simulink library "SimplusGT_2015a"  (R2015a)
settings: Solver=ode45  SolverMode=SingleTasking  StartTime=0.0  StopTime=10.0  RelTol=1e-3
undefined symbols (not defined in the file): ang_r, Cf, DiscIntNeverNeededParam, initial, Lc, Lf, m, OtherInputs, P_dc, Sbase, t0, Tm_pu, Ts, V, Vbase, w_droop, w_i, w_pll, w_tau, w_v, Wbase, wc, wfil, x0, Ybase, Zbase
libraries: powerlib x224, SimplexPS_2015a x6, SimplusGT_2015a x1
(part 4 of 5)

== system SimplusGT_2015a/Voltage Disturbance ==
  note: Model for a voltage disturbance.
      |
      | Author(s): Yitong Li
  vabc : Inport
  Controlled Voltage Source : powerlib/Electrical Sources/Controlled Voltage Source  Initialize=on  Source_Type=AC  Amplitude=0  Phase=0  Frequency=0  Measurements=None
  Controlled Voltage Source1 : powerlib/Electrical Sources/Controlled Voltage Source  Initialize=on  Source_Type=AC  Amplitude=0  Phase=0  Frequency=0  Measurements=None
  Controlled Voltage Source2 : powerlib/Electrical Sources/Controlled Voltage Source  Initialize=on  Source_Type=AC  Amplitude=0  Phase=0  Frequency=0  Measurements=None
  Demux : Demux  Outputs=3
  Gain : Gain  Gain=Vbase
  a+ : PMIOPort  Side=Right
  a- : PMIOPort  Port=2  Side=Left
  b+ : PMIOPort  Port=3  Side=Right
  b- : PMIOPort  Port=4  Side=Left
  c+ : PMIOPort  Port=5  Side=Right
  c- : PMIOPort  Port=6  Side=Left
  wires:
  vabc/1 -> Gain/1
  Demux/1 -> Controlled Voltage Source/1
  Demux/2 -> Controlled Voltage Source1/1
  Demux/3 -> Controlled Voltage Source2/1
  Gain/1 -> Demux/1
  connections:
  Controlled Voltage Source2/LConn1 -- c-/RConn1
  Controlled Voltage Source1/RConn1 -- b+/RConn1
  Controlled Voltage Source2/RConn1 -- c+/RConn1
  Controlled Voltage Source/RConn1 -- a+/RConn1
  Controlled Voltage Source/LConn1 -- a-/RConn1
  Controlled Voltage Source1/LConn1 -- b-/RConn1

== system SimplusGT_2015a/abc -> alpha//beta (Power-Invariant) ==
  note: Frame transformation from abc to alpha/beta.
      |
      | Author(s): Yitong Li
      |
      | Notes:
      |
      | The transformation is power-invariant.
  abc : Inport
  ->alpha : Fcn  Expr=u(1) - 1/2*u(2) - 1/2*u(3)
  ->beta : Fcn  Expr=0 + sqrt(3)/2*u(2) - sqrt(3)/2*u(3)
  Gain : Gain  Gain=sqrt(2/3)
  Mux2 : Mux  Inputs=2
  albe : Outport
  wires:
  abc/1 -> Gain/1
  Mux2/1 -> albe/1
  Gain/1 -> ->alpha/1, ->beta/1
  ->alpha/1 -> Mux2/1
  ->beta/1 -> Mux2/2

== system SimplusGT_2015a/abc -> alpha//beta//0 (Power-Invariant) ==
  note: Frame transformation from abc to alpha/beta/0.
      |
      | Author(s): Yitong Li
      |
      | Notes:
      |
      | The transformation is power-invariant.
  abc : Inport
  ->0 : Fcn  Expr=1/sqrt(2)*u(1) + 1/sqrt(2)*u(2) + 1/sqrt(2)*u(3)
  ->alpha : Fcn  Expr=u(1) - 1/2*u(2) - 1/2*u(3)
  ->beta : Fcn  Expr=0 + sqrt(3)/2*u(2) - sqrt(3)/2*u(3)
  Gain : Gain  Gain=sqrt(2/3)
  Mux2 : Mux  Inputs=3
  albe0 : Outport
  wires:
  ->beta/1 -> Mux2/2
  ->alpha/1 -> Mux2/1
  Gain/1 -> ->alpha/1, ->0/1, ->beta/1
  Mux2/1 -> albe0/1
  abc/1 -> Gain/1
  ->0/1 -> Mux2/3

== system SimplusGT_2015a/abc -> dq (Power-Invariant) ==
  note: Frame transformation from abc to dq.
      |
      | Author(s): Yitong Li
      |
      | Notes:
      |
      | The transformation is power-invariant.
      |
      | theta is the angle that d axis leads a axis.
      |
      | q axis leads d axis by 90 degrees.
  abc : Inport
  theta : Inport  Port=2
  ->d : Fcn  Expr=cos(u(4))*u(1) + cos(u(4)-2/3*pi)*u(2) + cos(u(4)-4/3*pi)*u(3)
  ->q : Fcn  Expr=-sin(u(4))*u(1) - sin(u(4)-2/3*pi)*u(2) - sin(u(4)-4/3*pi)*u(3)
  Gain : Gain  Gain=sqrt(2/3)
  Mux5 : Mux  Inputs=2
  Mux6 : Mux  Inputs=2
  dq : Outport
  wires:
  Mux5/1 -> ->q/1, ->d/1
  Mux6/1 -> dq/1
  ->q/1 -> Mux6/2
  theta/1 -> Mux5/2
  Gain/1 -> Mux5/1
  ->d/1 -> Mux6/1
  abc/1 -> Gain/1

== system SimplusGT_2015a/abc -> dq (Power-Invariant) (Complex Theta) ==
  abc : Inport
  theta+ : Inport  Port=2
  ->d : Fcn  Expr=cos(u(4))*u(1) + cos(u(4)-2/3*pi)*u(2) + cos(u(4)-4/3*pi)*u(3)
  ->q : Fcn  Expr=-sin(u(4))*u(1) - sin(u(4)-2/3*pi)*u(2) - sin(u(4)-4/3*pi)*u(3)
  Complex to Real-Imag : ComplexToRealImag
  Gain : Gain  Gain=sqrt(2/3)
  Math Function : Math  SaturateOnIntegerOverflow=on
  Mux5 : Mux  Inputs=2
  Mux6 : Mux  Inputs=2
  Product : Product
  dq : Outport
  wires:
  ->q/1 -> Mux6/2
  abc/1 -> Gain/1
  Mux5/1 -> ->q/1, ->d/1
  Mux6/1 -> dq/1
  ->d/1 -> Mux6/1
  theta+/1 -> Complex to Real-Imag/1
  Complex to Real-Imag/1 -> Mux5/2
  Complex to Real-Imag/2 -> Math Function/1
  Gain/1 -> Product/1
  Product/1 -> Mux5/1
  Math Function/1 -> Product/2

== system SimplusGT_2015a/abc -> dq0 (Power-Invariant) ==
  note: Frame transformation from abc to dq0.
      |
      | Author(s): Yitong Li
      |
      | Notes:
      |
      | The transformation is power-invariant.
      |
      | theta is the angle that dq axis leads abc axis, specifically, d axis leads a axis.
      |
      | q axis leads d axis by 90 degrees. b leads a axis 90 degrees. c leads b 90 degrees.
  abc : Inport
  theta : Inport  Port=2
  ->0 : Fcn  Expr=sqrt(2)/2*u(1) + sqrt(2)/2*u(2) + sqrt(2)/2*u(3)
  ->d : Fcn  Expr=cos(u(4))*u(1) + cos(u(4)-2/3*pi)*u(2) + cos(u(4)-4/3*pi)*u(3)
  ->q : Fcn  Expr=-sin(u(4))*u(1) - sin(u(4)-2/3*pi)*u(2) - sin(u(4)-4/3*pi)*u(3)
  Gain : Gain  Gain=sqrt(2/3)
  Mux1 : Mux  Inputs=2
  Mux2 : Mux  Inputs=3
  dq0 : Outport
  wires:
  ->d/1 -> Mux2/1
  ->q/1 -> Mux2/2
  Gain/1 -> Mux1/1
  abc/1 -> Gain/1
  theta/1 -> Mux1/2
  Mux1/1 -> ->0/1, ->d/1, ->q/1
  Mux2/1 -> dq0/1
  ->0/1 -> Mux2/3

== system SimplusGT_2015a/abc->dq (Power-Invariant) (theta_dq) ==
  abc : Inport
  theta_dq : Inport  Port=2
  ->d : Fcn  Expr=cos(u(4))*u(1) + cos(u(4)-2/3*pi)*u(2) + cos(u(4)-4/3*pi)*u(3)
  ->q : Fcn  Expr=-sin(u(4))*u(1) - sin(u(4)-2/3*pi)*u(2) - sin(u(4)-4/3*pi)*u(3)
  Demux : Demux  Outputs=2
  Gain : Gain  Gain=sqrt(2/3)
  Math Function : Math  SaturateOnIntegerOverflow=on
  Mux5 : Mux  Inputs=2
  Mux6 : Mux  Inputs=2
  Product : Product
  dq : Outport
  wires:
  Gain/1 -> Product/1
  Math Function/1 -> Product/2
  Mux6/1 -> dq/1
  Mux5/1 -> ->q/1, ->d/1
  ->d/1 -> Mux6/1
  Product/1 -> Mux5/1
  abc/1 -> Gain/1
  ->q/1 -> Mux6/2
  theta_dq/1 -> Demux/1
  Demux/1 -> Mux5/2
  Demux/2 -> Math Function/1

== system SimplusGT_2015a/alpha//beta -> abc (Power-Invariant) ==
  note: Frame transformation from alpha/beta to abc.
      |
      | Author(s): Yitong Li
      |
      | Notes:
      |
      | The transformation is power-invariant.
  albe : Inport
  ->a : Fcn  Expr=u(1) + 0
  ->b : Fcn  Expr=-1/2*u(1) + sqrt(3)/2*u(2)
  ->c : Fcn  Expr=-1/2*u(1) - sqrt(3)/2*u(2)
  Gain : Gain  Gain=sqrt(2/3)
  Mux2 : Mux  Inputs=3
  abc : Outport
  wires:
  Gain/1 -> ->a/1, ->c/1, ->b/1
  Mux2/1 -> abc/1
  ->c/1 -> Mux2/3
  ->b/1 -> Mux2/2
  ->a/1 -> Mux2/1
  albe/1 -> Gain/1

== system SimplusGT_2015a/alpha//beta -> dq ==
  note: Frame transformation from alpha/beta to dq.
      |
      | Author(s): Yitong Li
      |
      | Notes:
      |
      | theta is the angle that dq axis leads alpha/beta axis, specifically, d axis leads alpha axis.
  albe : Inport
  theta : Inport  Port=2
  ->d : Fcn  Expr=cos(u(3))*u(1) + sin(u(3))*u(2)
  ->q : Fcn  Expr=-sin(u(3))*u(1) + cos(u(3))*u(2)
  Mux5 : Mux  Inputs=2
  Mux6 : Mux  Inputs=2
  dq : Outport
  wires:
  Mux5/1 -> ->q/1, ->d/1
  albe/1 -> Mux5/1
  theta/1 -> Mux5/2
  Mux6/1 -> dq/1
  ->q/1 -> Mux6/2
  ->d/1 -> Mux6/1

== system SimplusGT_2015a/alpha//beta//0 -> abc (Power-Invariant) ==
  note: Frame transformation from alpha/beta0 to abc.
      |
      | Author(s): Yitong Li
      |
      | Notes:
      |
      | The transformation is power-invariant.
  albe0 : Inport
  ->a : Fcn  Expr=u(1) + 0 + 1/sqrt(2)*u(3)
  ->b : Fcn  Expr=-1/2*u(1) + sqrt(3)/2*u(2) + 1/sqrt(2)*u(3)
  ->c : Fcn  Expr=-1/2*u(1) - sqrt(3)/2*u(2) + 1/sqrt(2)*u(3)
  Gain : Gain  Gain=sqrt(2/3)
  Mux2 : Mux  Inputs=3
  abc : Outport
  wires:
  Gain/1 -> ->a/1, ->c/1, ->b/1
  ->c/1 -> Mux2/3
  albe0/1 -> Gain/1
  ->a/1 -> Mux2/1
  ->b/1 -> Mux2/2
  Mux2/1 -> abc/1

== system SimplusGT_2015a/dq -> abc (Power-Invariant) ==
  note: Frame transformation from dq to abc.
      |
      | Author(s): Yitong Li
      |
      | Notes:
      |
      | The transformation is power-invariant.
      |
      | theta is the angle that dq axis leads alpha/beta axis, specifically, d axis leads alpha axis.
  dq : Inport
  theta : Inport  Port=2
  ->a : Fcn  Expr=cos(u(3))*u(1) - sin(u(3))*u(2)
  ->b : Fcn  Expr=cos(u(3)-2/3*pi)*u(1) - sin(u(3)-2/3*pi)*u(2)
  ->c : Fcn  Expr=cos(u(3)-4/3*pi)*u(1) - sin(u(3)-4/3*pi)*u(2)
  Gain : Gain  Gain=sqrt(2/3)
  Mux5 : Mux  Inputs=2
  Mux6 : Mux  Inputs=3
  abc : Outport
  wires:
  theta/1 -> Mux5/2
  Mux5/1 -> ->c/1, ->a/1, ->b/1
  Mux6/1 -> abc/1
  ->c/1 -> Mux6/3
  dq/1 -> Gain/1
  Gain/1 -> Mux5/1
  ->a/1 -> Mux6/1
  ->b/1 -> Mux6/2

== system SimplusGT_2015a/dq -> abc (Power-Invariant) (Complex Theta) ==
  dq : Inport
  theta+ : Inport  Port=2
  ->a : Fcn  Expr=cos(u(3))*u(1) - sin(u(3))*u(2)
  ->b : Fcn  Expr=cos(u(3)-2/3*pi)*u(1) - sin(u(3)-2/3*pi)*u(2)
  ->c : Fcn  Expr=cos(u(3)-4/3*pi)*u(1) - sin(u(3)-4/3*pi)*u(2)
  Complex to Real-Imag : ComplexToRealImag
  Gain : Gain  Gain=sqrt(2/3)
  Gain1 : Gain  Gain=-1
  Math Function : Math  SaturateOnIntegerOverflow=on
  Mux5 : Mux  Inputs=2
  Mux6 : Mux  Inputs=3
  Product : Product
  abc : Outport
  wires:
  ->b/1 -> Mux6/2
  ->a/1 -> Mux6/1
  dq/1 -> Gain/1
  ->c/1 -> Mux6/3
  Mux6/1 -> abc/1
  Mux5/1 -> ->c/1, ->a/1, ->b/1
  theta+/1 -> Complex to Real-Imag/1
  Math Function/1 -> Product/2
  Complex to Real-Imag/1 -> Mux5/2
  Product/1 -> Mux5/1
  Gain/1 -> Product/1
  Complex to Real-Imag/2 -> Gain1/1
  Gain1/1 -> Math Function/1

== system SimplusGT_2015a/dq->abc (Power-Invariant) (theta_dq) ==
  dq : Inport
  theta_dq : Inport  Port=2
  ->a : Fcn  Expr=cos(u(3))*u(1) - sin(u(3))*u(2)
  ->b : Fcn  Expr=cos(u(3)-2/3*pi)*u(1) - sin(u(3)-2/3*pi)*u(2)
  ->c : Fcn  Expr=cos(u(3)-4/3*pi)*u(1) - sin(u(3)-4/3*pi)*u(2)
  Demux : Demux  Outputs=2
  Gain : Gain  Gain=sqrt(2/3)
  Gain1 : Gain  Gain=-1
  Math Function : Math  SaturateOnIntegerOverflow=on
  Mux5 : Mux  Inputs=2
  Mux6 : Mux  Inputs=3
  Product : Product
  abc : Outport
  wires:
  Mux6/1 -> abc/1
  Demux/1 -> Mux5/2
  Product/1 -> Mux5/1
  ->a/1 -> Mux6/1
  Gain1/1 -> Math Function/1
  Math Function/1 -> Product/2
  ->c/1 -> Mux6/3
  Mux5/1 -> ->c/1, ->a/1, ->b/1
  ->b/1 -> Mux6/2
  theta_dq/1 -> Demux/1
  Gain/1 -> Product/1
  dq/1 -> Gain/1
  Demux/2 -> Gain1/1

== system SimplusGT_2015a/dq0 -> abc (Power-Invariant) ==
  note: Frame transformation from dq0 to abc.
      |
      | Author(s): Yitong Li
      |
      | Notes:
      |
      | The transformation is power-invariant.
      |
      | theta is the angle that dq axis leads alpha/beta axis, specifically, d axis leads alpha axis.
  dq0 : Inport
  theta : Inport  Port=2
  ->a : Fcn  Expr=cos(u(4))*u(1) - sin(u(4))*u(2) + sqrt(2)/2*u(3)
  ->b : Fcn  Expr=cos(u(4)-2/3*pi)*u(1) - sin(u(4)-2/3*pi)*u(2) + sqrt(2)/2*u(3)
  ->c : Fcn  Expr=cos(u(4)-4/3*pi)*u(1) - sin(u(4)-4/3*pi)*u(2) + sqrt(2)/2*u(3)
  Gain : Gain  Gain=sqrt(2/3)
  Mux1 : Mux  Inputs=2
  Mux2 : Mux  Inputs=3
  abc : Outport
  wires:
  ->a/1 -> Mux2/1
  ->b/1 -> Mux2/2
  Gain/1 -> Mux1/1
  dq0/1 -> Gain/1
  theta/1 -> Mux1/2
  Mux1/1 -> ->c/1, ->a/1, ->b/1
  Mux2/1 -> abc/1
  ->c/1 -> Mux2/3

== system SimplusGT_2015a/x1y1 -> x2y2 ==
  note: Frame transformation from x1y1 to x2y2.
      |
      | Author(s): Yitong Li
      |
      | Notes:
      |
      | theta is the phase angle that coordinate 2 (axis) leads coordinate 1 (axis).
  x1y1 : Inport
  theta : Inport  Port=2
  ->x2 : Fcn  Expr=cos(u(3))*u(1) + sin(u(3))*u(2)
  ->y2 : Fcn  Expr=-sin(u(3))*u(1) + cos(u(3))*u(2)
  Mux5 : Mux  Inputs=2
  Mux6 : Mux  Inputs=2
  x2y2 : Outport
  wires:
  Mux6/1 -> x2y2/1
  Mux5/1 -> ->y2/1, ->x2/1
  theta/1 -> Mux5/2
  x1y1/1 -> Mux5/1
  ->y2/1 -> Mux6/2
  ->x2/1 -> Mux6/1

== system SimplusGT_2015a/x2y2 -> x1y1 ==
  note: Frame transformation from x2y2 to x1y1.
      |
      | Author(s): Yitong Li
      |
      | Notes:
      |
      | theta is the phase angle that coordinate 2 (axis) leads coordinate 1 (axis).
  x2y2 : Inport
  theta : Inport  Port=2
  ->x2 : Fcn  Expr=cos(u(3))*u(1) - sin(u(3))*u(2)
  ->y2 : Fcn  Expr=sin(u(3))*u(1) + cos(u(3))*u(2)
  Mux5 : Mux  Inputs=2
  Mux6 : Mux  Inputs=2
  x1y1 : Outport
  wires:
  theta/1 -> Mux5/2
  Mux6/1 -> x1y1/1
  Mux5/1 -> ->y2/1, ->x2/1
  x2y2/1 -> Mux5/1
  ->x2/1 -> Mux6/1
  ->y2/1 -> Mux6/2

== system SimplusGT_2015a/AC Infinite Bus (Current Type)/PQ Calculation (dq-Frame) ==
  note: Power calculation.
      |
      | Author(s): Yitong Li
      |
      | Notes:
      |
      | The calculation is done in dq frame.
  vdq : Inport
  idq : Inport  Port=2
  Mux : Mux  Inputs=2
  Mux1 : Mux  Inputs=2
  P = vd*id+vq*iq : Fcn  Expr=u[1]*u[3]+u[2]*u[4]
  Q = -vd*iq+vq*id : Fcn  Expr=-u[1]*u[4]+u[2]*u[3]
  pq : Outport
  wires:
  Q = -vd*iq+vq*id/1 -> Mux/2
  Mux1/1 -> Q = -vd*iq+vq*id/1, P = vd*id+vq*iq/1
  idq/1 -> Mux1/2
  vdq/1 -> Mux1/1
  P = vd*id+vq*iq/1 -> Mux/1
  Mux/1 -> pq/1

== system SimplusGT_2015a/AC Infinite Bus (Current Type)/abc -> dq (Power-Invariant) ==
  note: Frame transformation from abc to dq.
      |
      | Author(s): Yitong Li
      |
      | Notes:
      |
      | The transformation is power-invariant.
      |
      | theta is the angle that d axis leads a axis.
      |
      | q axis leads d axis by 90 degrees.
  abc : Inport
  theta : Inport  Port=2
  ->d : Fcn  Expr=cos(u(4))*u(1) + cos(u(4)-2/3*pi)*u(2) + cos(u(4)-4/3*pi)*u(3)
  ->q : Fcn  Expr=-sin(u(4))*u(1) - sin(u(4)-2/3*pi)*u(2) - sin(u(4)-4/3*pi)*u(3)
  Gain : Gain  Gain=sqrt(2/3)
  Mux5 : Mux  Inputs=2
  Mux6 : Mux  Inputs=2
  dq : Outport
  wires:
  Mux5/1 -> ->q/1, ->d/1
  Mux6/1 -> dq/1
  ->q/1 -> Mux6/2
  theta/1 -> Mux5/2
  Gain/1 -> Mux5/1
  ->d/1 -> Mux6/1
  abc/1 -> Gain/1

== system SimplusGT_2015a/AC Infinite Bus (Current Type)/dq -> abc (Power-Invariant) ==
  note: Frame transformation from dq to abc.
      |
      | Author(s): Yitong Li
      |
      | Notes:
      |
      | The transformation is power-invariant.
      |
      | theta is the angle that dq axis leads alpha/beta axis, specifically, d axis leads alpha axis.
  dq : Inport
  theta : Inport  Port=2
  ->a : Fcn  Expr=cos(u(3))*u(1) - sin(u(3))*u(2)
  ->b : Fcn  Expr=cos(u(3)-2/3*pi)*u(1) - sin(u(3)-2/3*pi)*u(2)
  ->c : Fcn  Expr=cos(u(3)-4/3*pi)*u(1) - sin(u(3)-4/3*pi)*u(2)
  Gain : Gain  Gain=sqrt(2/3)
  Mux5 : Mux  Inputs=2
  Mux6 : Mux  Inputs=3
  abc : Outport
  wires:
  theta/1 -> Mux5/2
  Mux5/1 -> ->c/1, ->a/1, ->b/1
  Mux6/1 -> abc/1
  ->c/1 -> Mux6/3
  dq/1 -> Gain/1
  Gain/1 -> Mux5/1
  ->a/1 -> Mux6/1
  ->b/1 -> Mux6/2

== system SimplusGT_2015a/AC Infinite Bus (Voltage Type)/PQ Calculation (dq-Frame)1 ==
  note: Power calculation.
      |
      | Author(s): Yitong Li
      |
      | Notes:
      |
      | The calculation is done in dq frame.
  vdq : Inport
  idq : Inport  Port=2
  Mux : Mux  Inputs=2
  Mux1 : Mux  Inputs=2
  P = vd*id+vq*iq : Fcn  Expr=u[1]*u[3]+u[2]*u[4]
  Q = -vd*iq+vq*id : Fcn  Expr=-u[1]*u[4]+u[2]*u[3]
  pq : Outport
  wires:
  Q = -vd*iq+vq*id/1 -> Mux/2
  Mux1/1 -> Q = -vd*iq+vq*id/1, P = vd*id+vq*iq/1
  idq/1 -> Mux1/2
  vdq/1 -> Mux1/1
  P = vd*id+vq*iq/1 -> Mux/1
  Mux/1 -> pq/1

== system SimplusGT_2015a/AC Infinite Bus (Voltage Type)/abc -> dq (Power-Invariant)1 ==
  note: Frame transformation from abc to dq.
      |
      | Author(s): Yitong Li
      |
      | Notes:
      |
      | The transformation is power-invariant.
      |
      | theta is the angle that d axis leads a axis.
      |
      | q axis leads d axis by 90 degrees.
  abc : Inport
  theta : Inport  Port=2
  ->d : Fcn  Expr=cos(u(4))*u(1) + cos(u(4)-2/3*pi)*u(2) + cos(u(4)-4/3*pi)*u(3)
  ->q : Fcn  Expr=-sin(u(4))*u(1) - sin(u(4)-2/3*pi)*u(2) - sin(u(4)-4/3*pi)*u(3)
  Gain : Gain  Gain=sqrt(2/3)
  Mux5 : Mux  Inputs=2
  Mux6 : Mux  Inputs=2
  dq : Outport
  wires:
  Mux5/1 -> ->q/1, ->d/1
  Mux6/1 -> dq/1
  ->q/1 -> Mux6/2
  theta/1 -> Mux5/2
  Gain/1 -> Mux5/1
  ->d/1 -> Mux6/1
  abc/1 -> Gain/1

== system SimplusGT_2015a/AC Infinite Bus (Voltage Type)/dq -> abc (Power-Invariant)1 ==
  note: Frame transformation from dq to abc.
      |
      | Author(s): Yitong Li
      |
      | Notes:
      |
      | The transformation is power-invariant.
      |
      | theta is the angle that dq axis leads alpha/beta axis, specifically, d axis leads alpha axis.
  dq : Inport
  theta : Inport  Port=2
  ->a : Fcn  Expr=cos(u(3))*u(1) - sin(u(3))*u(2)
  ->b : Fcn  Expr=cos(u(3)-2/3*pi)*u(1) - sin(u(3)-2/3*pi)*u(2)
  ->c : Fcn  Expr=cos(u(3)-4/3*pi)*u(1) - sin(u(3)-4/3*pi)*u(2)
  Gain : Gain  Gain=sqrt(2/3)
  Mux5 : Mux  Inputs=2
  Mux6 : Mux  Inputs=3
  abc : Outport
  wires:
  theta/1 -> Mux5/2
  Mux5/1 -> ->c/1, ->a/1, ->b/1
  Mux6/1 -> abc/1
  ->c/1 -> Mux6/3
  dq/1 -> Gain/1
  Gain/1 -> Mux5/1
  ->a/1 -> Mux6/1
  ->b/1 -> Mux6/2

== system SimplusGT_2015a/Frequency Droop (iDQ -> id)/x1y1 -> x2y2 ==
  note: Frame transformation from x1y1 to x2y2.
      |
      | Author(s): Yitong Li
      |
      | Notes:
      |
      | theta is the phase angle that coordinate 2 (axis) leads coordinate 1 (axis).
  x1y1 : Inport
  theta : Inport  Port=2
  ->x2 : Fcn  Expr=cos(u(3))*u(1) + sin(u(3))*u(2)
  ->y2 : Fcn  Expr=-sin(u(3))*u(1) + cos(u(3))*u(2)
  Mux5 : Mux  Inputs=2
  Mux6 : Mux  Inputs=2
  x2y2 : Outport
  wires:
  ->x2/1 -> Mux6/1
  ->y2/1 -> Mux6/2
  x1y1/1 -> Mux5/1
  theta/1 -> Mux5/2
  Mux5/1 -> ->x2/1, ->y2/1
  Mux6/1 -> x2y2/1

== system SimplusGT_2015a/Frequency Droop (iabc -> id)/abc -> dq (Power-Invariant) ==
  note: Frame transformation from abc to dq.
      |
      | Author(s): Yitong Li
      |
      | Notes:
      |
      | The transformation is power-invariant.
      |
      | theta is the angle that d axis leads a axis.
      |
      | q axis leads d axis by 90 degrees.
  abc : Inport
  theta : Inport  Port=2
  ->d : Fcn  Expr=cos(u(4))*u(1) + cos(u(4)-2/3*pi)*u(2) + cos(u(4)-4/3*pi)*u(3)
  ->q : Fcn  Expr=-sin(u(4))*u(1) - sin(u(4)-2/3*pi)*u(2) - sin(u(4)-4/3*pi)*u(3)
  Gain : Gain  Gain=sqrt(2/3)
  Mux5 : Mux  Inputs=2
  Mux6 : Mux  Inputs=2
  dq : Outport
  wires:
  abc/1 -> Gain/1
  ->d/1 -> Mux6/1
  Gain/1 -> Mux5/1
  theta/1 -> Mux5/2
  ->q/1 -> Mux6/2
  Mux6/1 -> dq/1
  Mux5/1 -> ->d/1, ->q/1

== system SimplusGT_2015a/Frequency Droop (iabc -> id+jiq)/abc -> dq (Power-Invariant)1 ==
  note: Frame transformation from abc to dq.
      |
      | Author(s): Yitong Li
      |
      | Notes:
      |
      | The transformation is power-invariant.
      |
      | theta is the angle that d axis leads a axis.
      |
      | q axis leads d axis by 90 degrees.
  abc : Inport
  theta : Inport  Port=2
  ->d : Fcn  Expr=cos(u(4))*u(1) + cos(u(4)-2/3*pi)*u(2) + cos(u(4)-4/3*pi)*u(3)
  ->q : Fcn  Expr=-sin(u(4))*u(1) - sin(u(4)-2/3*pi)*u(2) - sin(u(4)-4/3*pi)*u(3)
  Gain : Gain  Gain=sqrt(2/3)
  Mux5 : Mux  Inputs=2
  Mux6 : Mux  Inputs=2
  dq : Outport
  wires:
  abc/1 -> Gain/1
  ->d/1 -> Mux6/1
  Gain/1 -> Mux5/1
  theta/1 -> Mux5/2
  ->q/1 -> Mux6/2
  Mux6/1 -> dq/1
  Mux5/1 -> ->d/1, ->q/1

== system SimplusGT_2015a/Frequency Droop (iabc -> iq)/abc -> dq (Power-Invariant)1 ==
  note: Frame transformation from abc to dq.
      |
      | Author(s): Yitong Li
      |
      | Notes:
      |
      | The transformation is power-invariant.
      |
      | theta is the angle that d axis leads a axis.
      |
      | q axis leads d axis by 90 degrees.
  abc : Inport
  theta : Inport  Port=2
  ->d : Fcn  Expr=cos(u(4))*u(1) + cos(u(4)-2/3*pi)*u(2) + cos(u(4)-4/3*pi)*u(3)
  ->q : Fcn  Expr=-sin(u(4))*u(1) - sin(u(4)-2/3*pi)*u(2) - sin(u(4)-4/3*pi)*u(3)
  Gain : Gain  Gain=sqrt(2/3)
  Mux5 : Mux  Inputs=2
  Mux6 : Mux  Inputs=2
  dq : Outport
  wires:
  abc/1 -> Gain/1
  ->d/1 -> Mux6/1
  Gain/1 -> Mux5/1
  theta/1 -> Mux5/2
  ->q/1 -> Mux6/2
  Mux6/1 -> dq/1
  Mux5/1 -> ->d/1, ->q/1

== system SimplusGT_2015a/Grid-Following Voltage-Source Inverter (dq-Frame System Object)/PQ Calculation (dq-Frame)1 ==
  note: Power calculation.
      |
      | Author(s): Yitong Li
      |
      | Notes:
      |
      | The calculation is done in dq frame.
  vdq : Inport
  idq : Inport  Port=2
  Mux : Mux  Inputs=2
  Mux1 : Mux  Inputs=2
  P = vd*id+vq*iq : Fcn  Expr=u[1]*u[3]+u[2]*u[4]
  Q = -vd*iq+vq*id : Fcn  Expr=-u[1]*u[4]+u[2]*u[3]
  pq : Outport
  wires:
  Q = -vd*iq+vq*id/1 -> Mux/2
  Mux1/1 -> Q = -vd*iq+vq*id/1, P = vd*id+vq*iq/1
  idq/1 -> Mux1/2
  vdq/1 -> Mux1/1
  P = vd*id+vq*iq/1 -> Mux/1
  Mux/1 -> pq/1

== system SimplusGT_2015a/Grid-Following Voltage-Source Inverter (dq-Frame System Object)/abc -> dq (Power-Invariant)1 ==
  note: Frame transformation from abc to dq.
      |
      | Author(s): Yitong Li
      |
      | Notes:
      |
      | The transformation is power-invariant.
      |
      | theta is the angle that d axis leads a axis.
      |
      | q axis leads d axis by 90 degrees.
  abc : Inport
  theta : Inport  Port=2
  ->d : Fcn  Expr=cos(u(4))*u(1) + cos(u(4)-2/3*pi)*u(2) + cos(u(4)-4/3*pi)*u(3)
  ->q : Fcn  Expr=-sin(u(4))*u(1) - sin(u(4)-2/3*pi)*u(2) - sin(u(4)-4/3*pi)*u(3)
  Gain : Gain  Gain=sqrt(2/3)
  Mux5 : Mux  Inputs=2
  Mux6 : Mux  Inputs=2
  dq : Outport
  wires:
  Mux5/1 -> ->q/1, ->d/1
  Mux6/1 -> dq/1
  ->q/1 -> Mux6/2
  theta/1 -> Mux5/2
  Gain/1 -> Mux5/1
  ->d/1 -> Mux6/1
  abc/1 -> Gain/1

== system SimplusGT_2015a/Grid-Following Voltage-Source Inverter (dq-Frame System Object)/abc -> dq (Power-Invariant)2 ==
  note: Frame transformation from abc to dq.
      |
      | Author(s): Yitong Li
      |
      | Notes:
      |
      | The transformation is power-invariant.
      |
      | theta is the angle that d axis leads a axis.
      |
      | q axis leads d axis by 90 degrees.
  abc : Inport
  theta : Inport  Port=2
  ->d : Fcn  Expr=cos(u(4))*u(1) + cos(u(4)-2/3*pi)*u(2) + cos(u(4)-4/3*pi)*u(3)
  ->q : Fcn  Expr=-sin(u(4))*u(1) - sin(u(4)-2/3*pi)*u(2) - sin(u(4)-4/3*pi)*u(3)
  Gain : Gain  Gain=sqrt(2/3)
  Mux5 : Mux  Inputs=2
  Mux6 : Mux  Inputs=2
  dq : Outport
  wires:
  Mux5/1 -> ->q/1, ->d/1
  Mux6/1 -> dq/1
  ->q/1 -> Mux6/2
  theta/1 -> Mux5/2
  Gain/1 -> Mux5/1
  ->d/1 -> Mux6/1
  abc/1 -> Gain/1

== system SimplusGT_2015a/Grid-Following Voltage-Source Inverter (dq-Frame System Object)/dq -> abc (Power-Invariant)1 ==
  note: Frame transformation from dq to abc.
      |
      | Author(s): Yitong Li
      |
      | Notes:
      |
      | The transformation is power-invariant.
      |
      | theta is the angle that dq axis leads alpha/beta axis, specifically, d axis leads alpha axis.
  dq : Inport
  theta : Inport  Port=2
  ->a : Fcn  Expr=cos(u(3))*u(1) - sin(u(3))*u(2)
  ->b : Fcn  Expr=cos(u(3)-2/3*pi)*u(1) - sin(u(3)-2/3*pi)*u(2)
  ->c : Fcn  Expr=cos(u(3)-4/3*pi)*u(1) - sin(u(3)-4/3*pi)*u(2)
  Gain : Gain  Gain=sqrt(2/3)
  Mux5 : Mux  Inputs=2
  Mux6 : Mux  Inputs=3
  abc : Outport
  wires:
  theta/1 -> Mux5/2
  Mux5/1 -> ->c/1, ->a/1, ->b/1
  Mux6/1 -> abc/1
  ->c/1 -> Mux6/3
  dq/1 -> Gain/1
  Gain/1 -> Mux5/1
  ->a/1 -> Mux6/1
  ->b/1 -> Mux6/2

== system SimplusGT_2015a/Grid-Following Inverter (Simulink Block)/Current Controller ==
  iIdq* : Inport
  iIdq : Inport  Port=2
  vdq : Inport  Port=3
  enable : Inport  Port=4
  Constant : Constant  Value=Kcd
  Demux1 : Demux  Outputs=2
  Demux2 : Demux  Outputs=2
  Demux3 : Demux  Outputs=2
  Mux : Mux  Inputs=2
  PI-DT-Estimated d : Subsystem  mask{Lf=Lf, Kg=Kg, Kp=Kp, Ki=Ki, xmax=vdmax, xmin=-vdmax, Ts=Ts}
      mask prompts: Lf "Inductance"; Kg "Estimator Gain"; Kp "Proportional Gain"; Ki "Integral Gain"; xmax "Upper Limit"; xmin "Lower Limit"; Ts "Sampling Time"
  PI-DT-Estimated q : Subsystem  mask{Lf=Lf, Kg=Kg, Kp=Kp, Ki=Ki, xmax=vqmax, xmin=-vqmax, Ts=Ts}
      mask prompts: Lf "Inductance"; Kg "Estimator Gain"; Kp "Proportional Gain"; Ki "Integral Gain"; xmax "Upper Limit"; xmin "Lower Limit"; Ts "Sampling Time"
  Product : Product
  Product1 : Product
  sum_d : Sum  Inputs=+-
  sum_q : Sum
  wLd : Gain  Gain=Wbase*Lf
  wLq : Gain  Gain=Wbase*Lf
  vidq* : Outport
  wires:
  sum_d/1 -> Mux/1
  sum_q/1 -> Mux/2
  iIdq/1 -> Demux1/1
  Demux1/1 -> wLd/1, PI-DT-Estimated d/4(actual)
  Demux1/2 -> PI-DT-Estimated q/1(actual), wLq/1
  Mux/1 -> vidq*/1
  PI-DT-Estimated d/1(Out) -> sum_d/1
  vdq/1 -> Demux3/1
  PI-DT-Estimated q/1(Out) -> sum_q/2
  Demux3/2 -> PI-DT-Estimated q/2(initial)
  Demux3/1 -> PI-DT-Estimated d/3(initial)
  iIdq*/1 -> Demux2/1
  Demux2/1 -> PI-DT-Estimated d/2(reference)
  Demux2/2 -> PI-DT-Estimated q/3(reference)
  enable/1 -> PI-DT-Estimated q/4(enable), PI-DT-Estimated d/1(enable)
  wLd/1 -> Product/1
  Product/1 -> sum_q/1
  wLq/1 -> Product1/2
  Product1/1 -> sum_d/2
  Constant/1 -> Product/2, Product1/1

== system SimplusGT_2015a/Grid-Following Inverter (Simulink Block)/LCL Filter ==
  note: Model for a LCL filter.
      |
      | Author(s): Yitong Li
      |
      | Notes:
      |
      | vi is the converter side voltage, and vg is the grid side voltage.
  Bus Creator : BusCreator  Inputs=5
  "LL -> LN1" : Subsystem  AncestorBlock=|
      | SimplusGT/Grid-Forming Inverter
      | (Simulink Block)/LCL Filter/LL -> LN1
  "LL -> LN2" : Subsystem  AncestorBlock=|
      | SimplusGT/Grid-Forming Inverter
      | (Simulink Block)/LCL Filter/LL -> LN1
  Mux{,1..4} (5 alike) : Mux  Inputs=3
  Three-Phase Series RLC Branch : powerlib/Elements/Three-Phase Series RLC Branch  LConnTagsString=A|B|C  RConnTagsString=A|B|C  BranchType=RL  Resistance=Rf  Inductance=Lf  Capacitance=1e-6  Measurements=None
  Three-Phase Series RLC Branch1 : powerlib/Elements/Three-Phase Series RLC Branch  LConnTagsString=A|B|C  RConnTagsString=A|B|C  BranchType=RL  Resistance=Rc  Inductance=Lc  Capacitance=1e-6  Measurements=None
  Three-Phase Series RLC Branch2 : powerlib/Elements/Three-Phase Series RLC Branch  LConnTagsString=A|B|C  RConnTagsString=A|B|C  BranchType=RC  Resistance=Rd  Inductance=Lc  Capacitance=Cf  Measurements=None
  Vab : powerlib/Measurements/Voltage Measurement  PhasorSimulation=off  OutputType=Complex  PSBequivalent=0
  Vab1 : powerlib/Measurements/Voltage Measurement  PhasorSimulation=off  OutputType=Complex  PSBequivalent=0
  Vbc : powerlib/Measurements/Voltage Measurement  PhasorSimulation=off  OutputType=Complex  PSBequivalent=0
  Vbc1 : powerlib/Measurements/Voltage Measurement  PhasorSimulation=off  OutputType=Complex  PSBequivalent=0
  Vca : powerlib/Measurements/Voltage Measurement  PhasorSimulation=off  OutputType=Complex  PSBequivalent=0
  Vca1 : powerlib/Measurements/Voltage Measurement  PhasorSimulation=off  OutputType=Complex  PSBequivalent=0
  iga : powerlib/Measurements/Current Measurement  PhasorSimulation=off  OutputType=Complex  PSBequivalent=0
  igb : powerlib/Measurements/Current Measurement  PhasorSimulation=off  OutputType=Complex  PSBequivalent=0
  igc : powerlib/Measurements/Current Measurement  PhasorSimulation=off  OutputType=Complex  PSBequivalent=0
  ila : powerlib/Measurements/Current Measurement  PhasorSimulation=off  OutputType=Complex  PSBequivalent=0
  ilb : powerlib/Measurements/Current Measurement  PhasorSimulation=off  OutputType=Complex  PSBequivalent=0
  ilc : powerlib/Measurements/Current Measurement  PhasorSimulation=off  OutputType=Complex  PSBequivalent=0
  vca measure : powerlib/Measurements/Voltage Measurement  PhasorSimulation=off  OutputType=Complex  PSBequivalent=0
  vcb measure : powerlib/Measurements/Voltage Measurement  PhasorSimulation=off  OutputType=Complex  PSBequivalent=0
  vcc measure : powerlib/Measurements/Voltage Measurement  PhasorSimulation=off  OutputType=Complex  PSBequivalent=0
  via : PMIOPort  Side=Left
  vib : PMIOPort  Port=2  Side=Left
  vic : PMIOPort  Port=3  Side=Left
  vga : PMIOPort  Port=4  Side=Right
  vgb : PMIOPort  Port=5  Side=Right
  vgc : PMIOPort  Port=6  Side=Right
  N : PMIOPort  Port=7  Side=Left
  m : Outport
  wires:
  [igabc] -> Bus Creator/5  "igabc"
  [ilabc] -> Bus Creator/4  "ilabc"
  [vgabc] -> Bus Creator/3  "vgabc"
  [vcabc] -> Bus Creator/2  "vcabc"
  [viabc] -> Bus Creator/1  "viabc"
  "LL -> LN2"/1(Out1) -> [viabc]
  Vab1/1 -> Mux1/1
  Mux1/1 -> "LL -> LN2"/1(In1)
  Vca1/1 -> Mux1/3
  Vbc1/1 -> Mux1/2
  Mux3/1 -> [vcabc]
  "LL -> LN1"/1(Out1) -> [vgabc]
  Bus Creator/1 -> m/1
  Mux2/1 -> [ilabc]
  Vbc/1 -> Mux/2
  ilc/1 -> Mux2/3
  Vca/1 -> Mux/3
  iga/1 -> Mux4/1
  igb/1 -> Mux4/2
  vcb measure/1 -> Mux3/2
  vca measure/1 -> Mux3/1
  Mux/1 -> "LL -> LN1"/1(In1)
  Vab/1 -> Mux/1
  vcc measure/1 -> Mux3/3
  igc/1 -> Mux4/3
  ila/1 -> Mux2/1
  ilb/1 -> Mux2/2
  Mux4/1 -> [igabc]
  connections:
  Three-Phase Series RLC Branch/RConn3 -- ilc/LConn1
  Three-Phase Series RLC Branch/RConn2 -- ilb/LConn1
  Three-Phase Series RLC Branch/RConn1 -- ila/LConn1
  Three-Phase Series RLC Branch1/RConn3 -- igc/LConn1
  Three-Phase Series RLC Branch1/RConn1 -- iga/LConn1
  vga/RConn1 -- iga/RConn1 -- Vca/LConn2 -- Vab/LConn1
  Three-Phase Series RLC Branch2/LConn1 -- vca measure/LConn1 -- Three-Phase Series RLC Branch1/LConn1 -- ila/RConn1
  Three-Phase Series RLC Branch2/LConn2 -- vcb measure/LConn1 -- Three-Phase Series RLC Branch1/LConn2 -- ilb/RConn1
  vgb/RConn1 -- igb/RConn1 -- Vab/LConn2 -- Vbc/LConn1
  Three-Phase Series RLC Branch1/RConn2 -- igb/LConn1
  vcc measure/LConn1 -- Three-Phase Series RLC Branch2/LConn3 -- ilc/RConn1 -- Three-Phase Series RLC Branch1/LConn3
  Three-Phase Series RLC Branch/LConn1 -- via/RConn1 -- Vca1/LConn2 -- Vab1/LConn1
  vib/RConn1 -- Vab1/LConn2 -- Vbc1/LConn1 -- Three-Phase Series RLC Branch/LConn2
  Three-Phase Series RLC Branch/LConn3 -- vic/RConn1 -- Vbc1/LConn2 -- Vca1/LConn1
  vgc/RConn1 -- igc/RConn1 -- Vbc/LConn2 -- Vca/LConn1
  vcb measure/LConn2 -- vca measure/LConn2 -- vcc measure/LConn2 -- Three-Phase Series RLC Branch2/RConn3 -- N/RConn1 -- Three-Phase Series RLC Branch2/RConn2 -- Three-Phase Series RLC Branch2/RConn1

== system SimplusGT_2015a/Grid-Following Inverter (Simulink Block)/PLL (vabc -> vq) ==
  note: Phase lock loop (PLL)
      |
      | Author(s): Yitong Li
      |
      | Notes:
      |
      | vq is fed into the PI controller of the PLL.
  note: Gpll
  note: Measurement
  vabc : Inport
  Constant1 : Constant
  Constant2 : Constant  Value=theta0
  Constant3 : Constant
  Constant4 : Constant  Value=2*pi
  Constant6 : Constant  Value=0
  Demux1 : Demux  Outputs=2
  Discrete PI : Subsystem  AncestorBlock=SimplusGT/Discrete PI  mask{Kp=w_pll, Ki=w_pll*w_pll/4, xmax=inf, xmin=-inf, Ts=Ts}
      mask prompts: Kp "Proportional Gain"; Ki "Integral Gain"; xmax "Upper Limit"; xmin "Lower Limit"; Ts "Sampling Time"
  Discrete-Time Integrator : DiscreteIntegrator  SampleTime=Ts  ICPrevOutput=DiscIntNeverNeededParam  ICPrevScaledInput=DiscIntNeverNeededParam
  Filter p : DiscreteTransferFcn  Numerator=w_tau*Ts  Denominator=[1 ((w_tau*Ts)-1)]  SampleTime=Ts
  Gain1 : Gain  Gain=Wbase
  Gain2 : Gain  Gain=1/Vbase
  Gain4 : Gain  Gain=1/Wbase
  Gain5 : Gain  Gain=1/pi
  Math Function1 : Math  Operator=mod  SaturateOnIntegerOverflow=on
  Mux : Mux  Inputs=2
  Scope : Scope  NumInputPorts=4
      settings: TimeRange=auto  MaxDataPoints=5000  SaveToWorkspace=off  SaveName=ScopeData3  YMin=-0.01955~-0.01955~-0.01955~-0.01955  YMax=0.17599~0.17599~0.17599~0.17599  SampleTime=-1
  Sum : Sum
  Sum1 : Sum
  "abc -> dq (Power-Invariant)" : Subsystem  AncestorBlock=|
      | SimplusGT/abc -> dq
      | (Power-Invariant)
  w : Outport
  theta : Outport  Port=2
  vdq : Outport  Port=3
  wires:
  Math Function1/1 -> theta/1, [theta], "abc -> dq (Power-Invariant)"/2(theta)
  Constant3/1 -> Gain1/1
  Demux1/1 -> [vd]
  [theta] -> Mux/2  "theta"
  Gain5/1 -> Scope/4
  [vd] -> Scope/1  "vd"
  [theta0] -> Mux/1  "theta0"
  [w] -> Gain4/1  "w"
  Gain4/1 -> Scope/3
  Mux/1 -> Gain5/1
  [vq] -> Scope/2  "vq"
  Filter p/1 -> Discrete PI/2(reference)
  Constant2/1 -> Sum1/2, [theta0]
  Sum1/1 -> Math Function1/1
  Discrete-Time Integrator/1 -> Sum1/1
  Gain1/1 -> Sum/2
  Sum/1 -> Discrete-Time Integrator/1, w/1, [w]
  Discrete PI/1(Out) -> Sum/1
  Constant1/1 -> Discrete PI/1(enable)
  Constant6/1 -> Discrete PI/3(initial), Discrete PI/4(actual)
  Demux1/2 -> Gain2/1, [vq]
  Gain2/1 -> Filter p/1
  Constant4/1 -> Math Function1/2
  "abc -> dq (Power-Invariant)"/1(dq) -> Demux1/1, vdq/1
  vabc/1 -> "abc -> dq (Power-Invariant)"/1(abc)

== system SimplusGT_2015a/Grid-Following Inverter (Simulink Block)/PQ Calculation (dq-Frame)1 ==
  note: Power calculation.
      |
      | Author(s): Yitong Li
      |
      | Notes:
      |
      | The calculation is done in dq frame.
  vdq : Inport
  idq : Inport  Port=2
  Mux : Mux  Inputs=2
  Mux1 : Mux  Inputs=2
  P = vd*id+vq*iq : Fcn  Expr=u[1]*u[3]+u[2]*u[4]
  Q = -vd*iq+vq*id : Fcn  Expr=-u[1]*u[4]+u[2]*u[3]
  pq : Outport
  wires:
  Q = -vd*iq+vq*id/1 -> Mux/2
  Mux1/1 -> Q = -vd*iq+vq*id/1, P = vd*id+vq*iq/1
  idq/1 -> Mux1/2
  vdq/1 -> Mux1/1
  P = vd*id+vq*iq/1 -> Mux/1
  Mux/1 -> pq/1

== system SimplusGT_2015a/Grid-Following Inverter (Simulink Block)/abc -> dq (Power-Invariant)1 ==
  note: Frame transformation from abc to dq.
      |
      | Author(s): Yitong Li
      |
      | Notes:
      |
      | The transformation is power-invariant.
      |
      | theta is the angle that d axis leads a axis.
      |
      | q axis leads d axis by 90 degrees.
  abc : Inport
  theta : Inport  Port=2
  ->d : Fcn  Expr=cos(u(4))*u(1) + cos(u(4)-2/3*pi)*u(2) + cos(u(4)-4/3*pi)*u(3)
  ->q : Fcn  Expr=-sin(u(4))*u(1) - sin(u(4)-2/3*pi)*u(2) - sin(u(4)-4/3*pi)*u(3)
  Gain : Gain  Gain=sqrt(2/3)
  Mux5 : Mux  Inputs=2
  Mux6 : Mux  Inputs=2
  dq : Outport
  wires:
  Mux5/1 -> ->q/1, ->d/1
  Mux6/1 -> dq/1
  ->q/1 -> Mux6/2
  theta/1 -> Mux5/2
  Gain/1 -> Mux5/1
  ->d/1 -> Mux6/1
  abc/1 -> Gain/1

== system SimplusGT_2015a/Grid-Following Inverter (Simulink Block)/abc -> dq (Power-Invariant)2 ==
  note: Frame transformation from abc to dq.
      |
      | Author(s): Yitong Li
      |
      | Notes:
      |
      | The transformation is power-invariant.
      |
      | theta is the angle that d axis leads a axis.
      |
      | q axis leads d axis by 90 degrees.
  abc : Inport
  theta : Inport  Port=2
  ->d : Fcn  Expr=cos(u(4))*u(1) + cos(u(4)-2/3*pi)*u(2) + cos(u(4)-4/3*pi)*u(3)
  ->q : Fcn  Expr=-sin(u(4))*u(1) - sin(u(4)-2/3*pi)*u(2) - sin(u(4)-4/3*pi)*u(3)
  Gain : Gain  Gain=sqrt(2/3)
  Mux5 : Mux  Inputs=2
  Mux6 : Mux  Inputs=2
  dq : Outport
  wires:
  Mux5/1 -> ->q/1, ->d/1
  Mux6/1 -> dq/1
  ->q/1 -> Mux6/2
  theta/1 -> Mux5/2
  Gain/1 -> Mux5/1
  ->d/1 -> Mux6/1
  abc/1 -> Gain/1

== system SimplusGT_2015a/Grid-Following Inverter (Simulink Block)/abc -> dq (Power-Invariant)4 ==
  note: Frame transformation from abc to dq.
      |
      | Author(s): Yitong Li
      |
      | Notes:
      |
      | The transformation is power-invariant.
      |
      | theta is the angle that d axis leads a axis.
      |
      | q axis leads d axis by 90 degrees.
  abc : Inport
  theta : Inport  Port=2
  ->d : Fcn  Expr=cos(u(4))*u(1) + cos(u(4)-2/3*pi)*u(2) + cos(u(4)-4/3*pi)*u(3)
  ->q : Fcn  Expr=-sin(u(4))*u(1) - sin(u(4)-2/3*pi)*u(2) - sin(u(4)-4/3*pi)*u(3)
  Gain : Gain  Gain=sqrt(2/3)
  Mux5 : Mux  Inputs=2
  Mux6 : Mux  Inputs=2
  dq : Outport
  wires:
  Mux5/1 -> ->q/1, ->d/1
  Mux6/1 -> dq/1
  ->q/1 -> Mux6/2
  theta/1 -> Mux5/2
  Gain/1 -> Mux5/1
  ->d/1 -> Mux6/1
  abc/1 -> Gain/1

== system SimplusGT_2015a/Grid-Following Inverter (Simulink Block)/dq -> abc (Power-Invariant)1 ==
  note: Frame transformation from dq to abc.
      |
      | Author(s): Yitong Li
      |
      | Notes:
      |
      | The transformation is power-invariant.
      |
      | theta is the angle that dq axis leads alpha/beta axis, specifically, d axis leads alpha axis.
  dq : Inport
  theta : Inport  Port=2
  ->a : Fcn  Expr=cos(u(3))*u(1) - sin(u(3))*u(2)
  ->b : Fcn  Expr=cos(u(3)-2/3*pi)*u(1) - sin(u(3)-2/3*pi)*u(2)
  ->c : Fcn  Expr=cos(u(3)-4/3*pi)*u(1) - sin(u(3)-4/3*pi)*u(2)
  Gain : Gain  Gain=sqrt(2/3)
  Mux5 : Mux  Inputs=2
  Mux6 : Mux  Inputs=3
  abc : Outport
  wires:
  theta/1 -> Mux5/2
  Mux5/1 -> ->c/1, ->a/1, ->b/1
  Mux6/1 -> abc/1
  ->c/1 -> Mux6/3
  dq/1 -> Gain/1
  Gain/1 -> Mux5/1
  ->a/1 -> Mux6/1
  ->b/1 -> Mux6/2

== system SimplusGT_2015a/Grid-Forming Voltage-Source Inverter (dq-Frame System Object)/PQ Calculation (dq-Frame) ==
  note: Power calculation.
      |
      | Author(s): Yitong Li
      |
      | Notes:
      |
      | The calculation is done in dq frame.
  vdq : Inport
  idq : Inport  Port=2
  Mux : Mux  Inputs=2
  Mux1 : Mux  Inputs=2
  P = vd*id+vq*iq : Fcn  Expr=u[1]*u[3]+u[2]*u[4]
  Q = -vd*iq+vq*id : Fcn  Expr=-u[1]*u[4]+u[2]*u[3]
  pq : Outport
  wires:
  Mux/1 -> pq/1
  P = vd*id+vq*iq/1 -> Mux/1
  vdq/1 -> Mux1/1
  idq/1 -> Mux1/2
  Mux1/1 -> P = vd*id+vq*iq/1, Q = -vd*iq+vq*id/1
  Q = -vd*iq+vq*id/1 -> Mux/2

== system SimplusGT_2015a/Grid-Forming Voltage-Source Inverter (dq-Frame System Object)/abc -> dq (Power-Invariant) ==
  note: Frame transformation from abc to dq.
      |
      | Author(s): Yitong Li
      |
      | Notes:
      |
      | The transformation is power-invariant.
      |
      | theta is the angle that d axis leads a axis.
      |
      | q axis leads d axis by 90 degrees.
  abc : Inport
  theta : Inport  Port=2
  ->d : Fcn  Expr=cos(u(4))*u(1) + cos(u(4)-2/3*pi)*u(2) + cos(u(4)-4/3*pi)*u(3)
  ->q : Fcn  Expr=-sin(u(4))*u(1) - sin(u(4)-2/3*pi)*u(2) - sin(u(4)-4/3*pi)*u(3)
  Gain : Gain  Gain=sqrt(2/3)
  Mux5 : Mux  Inputs=2
  Mux6 : Mux  Inputs=2
  dq : Outport
  wires:
  abc/1 -> Gain/1
  ->d/1 -> Mux6/1
  Gain/1 -> Mux5/1
  theta/1 -> Mux5/2
  ->q/1 -> Mux6/2
  Mux6/1 -> dq/1
  Mux5/1 -> ->d/1, ->q/1

== system SimplusGT_2015a/Grid-Forming Voltage-Source Inverter (dq-Frame System Object)/abc -> dq (Power-Invariant)1 ==
  note: Frame transformation from abc to dq.
      |
      | Author(s): Yitong Li
      |
      | Notes:
      |
      | The transformation is power-invariant.
      |
      | theta is the angle that d axis leads a axis.
      |
      | q axis leads d axis by 90 degrees.
  abc : Inport
  theta : Inport  Port=2
  ->d : Fcn  Expr=cos(u(4))*u(1) + cos(u(4)-2/3*pi)*u(2) + cos(u(4)-4/3*pi)*u(3)
  ->q : Fcn  Expr=-sin(u(4))*u(1) - sin(u(4)-2/3*pi)*u(2) - sin(u(4)-4/3*pi)*u(3)
  Gain : Gain  Gain=sqrt(2/3)
  Mux5 : Mux  Inputs=2
  Mux6 : Mux  Inputs=2
  dq : Outport
  wires:
  abc/1 -> Gain/1
  ->d/1 -> Mux6/1
  Gain/1 -> Mux5/1
  theta/1 -> Mux5/2
  ->q/1 -> Mux6/2
  Mux6/1 -> dq/1
  Mux5/1 -> ->d/1, ->q/1

== system SimplusGT_2015a/Grid-Forming Voltage-Source Inverter (dq-Frame System Object)/dq -> abc (Power-Invariant) ==
  note: Frame transformation from dq to abc.
      |
      | Author(s): Yitong Li
      |
      | Notes:
      |
      | The transformation is power-invariant.
      |
      | theta is the angle that dq axis leads alpha/beta axis, specifically, d axis leads alpha axis.
  dq : Inport
  theta : Inport  Port=2
  ->a : Fcn  Expr=cos(u(3))*u(1) - sin(u(3))*u(2)
  ->b : Fcn  Expr=cos(u(3)-2/3*pi)*u(1) - sin(u(3)-2/3*pi)*u(2)
  ->c : Fcn  Expr=cos(u(3)-4/3*pi)*u(1) - sin(u(3)-4/3*pi)*u(2)
  Gain : Gain  Gain=sqrt(2/3)
  Mux5 : Mux  Inputs=2
  Mux6 : Mux  Inputs=3
  abc : Outport
  wires:
  ->b/1 -> Mux6/2
  ->a/1 -> Mux6/1
  Gain/1 -> Mux5/1
  dq/1 -> Gain/1
  ->c/1 -> Mux6/3
  Mux6/1 -> abc/1
  Mux5/1 -> ->b/1, ->a/1, ->c/1
  theta/1 -> Mux5/2

== system SimplusGT_2015a/Grid-Forming Inverter (Simulink Block)/Current Controller ==
  iIdq* : Inport
  iIdq : Inport  Port=2
  vdq : Inport  Port=3
  enable : Inport  Port=4
  Constant : Constant  Value=Kcd
  Demux1 : Demux  Outputs=2
  Demux2 : Demux  Outputs=2
  Demux3 : Demux  Outputs=2
  Mux : Mux  Inputs=2
  PI-DT-Estimated d : Subsystem  mask{Lf=Lf, Kg=Kg, Kp=Kp, Ki=Ki, xmax=xdmax, xmin=-xdmax, Ts=Ts}
      mask prompts: Lf "Inductance"; Kg "Estimator Gain"; Kp "Proportional Gain"; Ki "Integral Gain"; xmax "Upper Limit"; xmin "Lower Limit"; Ts "Sampling Time"
  PI-DT-Estimated q : Subsystem  mask{Lf=Lf, Kg=Kg, Kp=Kp, Ki=Ki, xmax=xqmax, xmin=-xqmax, Ts=Ts}
      mask prompts: Lf "Inductance"; Kg "Estimator Gain"; Kp "Proportional Gain"; Ki "Integral Gain"; xmax "Upper Limit"; xmin "Lower Limit"; Ts "Sampling Time"
  Product : Product
  Product1 : Product
  sum_d : Sum  Inputs=+-
  sum_q : Sum
  wLd : Gain  Gain=Wbase*Lf
  wLq : Gain  Gain=Wbase*Lf
  vidq* : Outport
  wires:
  sum_d/1 -> Mux/1
  sum_q/1 -> Mux/2
  iIdq/1 -> Demux1/1
  Demux1/1 -> wLd/1, PI-DT-Estimated d/4(actual)
  Demux1/2 -> PI-DT-Estimated q/1(actual), wLq/1
  Mux/1 -> vidq*/1
  PI-DT-Estimated d/1(Out) -> sum_d/1
  vdq/1 -> Demux3/1
  PI-DT-Estimated q/1(Out) -> sum_q/2
  Demux3/2 -> PI-DT-Estimated q/2(initial)
  Demux3/1 -> PI-DT-Estimated d/3(initial)
  iIdq*/1 -> Demux2/1
  Demux2/1 -> PI-DT-Estimated d/2(reference)
  Demux2/2 -> PI-DT-Estimated q/3(reference)
  enable/1 -> PI-DT-Estimated q/4(enable), PI-DT-Estimated d/1(enable)
  wLd/1 -> Product/1
  Product/1 -> sum_q/1
  wLq/1 -> Product1/2
  Product1/1 -> sum_d/2
  Constant/1 -> Product/2, Product1/1

== system SimplusGT_2015a/Grid-Forming Inverter (Simulink Block)/Frequency Droop (iabc -> id) ==
  note: id-frequency droop controller
      |
      | Author(s): Yitong Li
      |
      | Notes:
      |
      | The current reference should be in source convention.
      |
      | It is a id-frequency droop controller rather than a power-frequency droop controller.
  note: Measurement
  iabc : Inport
  Constant : Constant  Value=w0
  Constant2 : Constant  Value=theta0
  Constant4 : Constant  Value=2*pi
  Constant6 : Constant  Value=i0
  Demux1 : Demux  Outputs=2
  Discrete-Time Integrator : DiscreteIntegrator  SampleTime=Ts  ICPrevOutput=DiscIntNeverNeededParam  ICPrevScaledInput=DiscIntNeverNeededParam
  Filter p : DiscreteTransferFcn  Numerator=w_tau*Ts  Denominator=[1 ((w_tau*Ts)-1)]  SampleTime=Ts
  Gain1 : Gain  Gain=1/(Sbase/Vbase)
  Gain2 : Gain  Gain=m
  Gain3 : Gain  Gain=Wbase
  Gain4 : Gain  Gain=1/Wbase
  Gain5 : Gain  Gain=1/pi
  Math Function1 : Math  Operator=mod  SaturateOnIntegerOverflow=on
  Mux : Mux  Inputs=2
  Scope : Scope  NumInputPorts=4
      settings: TimeRange=auto  MaxDataPoints=5000  SaveToWorkspace=off  YMin=-0.01955~-0.01955~-0.01955~-0.01955  YMax=0.17599~0.17599~0.17599~0.17599  SampleTime=-1
  Sum : Sum
  Sum1 : Sum
  Sum2 : Sum  Inputs=+-
  "abc -> dq (Power-Invariant)" : Subsystem  AncestorBlock=|
      | SimplusGT/abc -> dq
      | (Power-Invariant)
  w : Outport
  theta : Outport  Port=2
  idq : Outport  Port=3
  wires:
  Gain4/1 -> Scope/3
  [w] -> Gain4/1  "w"
  Demux1/2 -> [iq]
  [theta] -> Mux/2  "theta"
  Mux/1 -> Gain5/1  "theta"
  [id] -> Scope/1  "id"
  [theta0] -> Mux/1  "theta"
  [iq] -> Scope/2  "iq"
  Gain5/1 -> Scope/4
  Demux1/1 -> [id], Gain1/1  "id"
  Gain3/1 -> Discrete-Time Integrator/1, w/1, [w]
  Sum/1 -> Gain3/1
  Sum2/1 -> Gain2/1
  Constant6/1 -> Sum2/1
  Gain1/1 -> Filter p/1
  iabc/1 -> "abc -> dq (Power-Invariant)"/1(abc)
  Constant4/1 -> Math Function1/2
  "abc -> dq (Power-Invariant)"/1(dq) -> Demux1/1, idq/1
  Constant/1 -> Sum/2
  Filter p/1 -> Sum2/2
  Discrete-Time Integrator/1 -> Sum1/1
  Gain2/1 -> Sum/1
  Math Function1/1 -> theta/1, [theta], "abc -> dq (Power-Invariant)"/2(theta)
  Constant2/1 -> [theta0], Sum1/2
  Sum1/1 -> Math Function1/1

== system SimplusGT_2015a/Grid-Forming Inverter (Simulink Block)/LCL Filter ==
  note: Model for a LCL filter.
      |
      | Author(s): Yitong Li
      |
      | Notes:
      |
      | vi is the converter side voltage, and vg is the grid side voltage.
  Bus Creator : BusCreator  Inputs=5
  "LL -> LN" : Subsystem  AncestorBlock=SimplusGT/LL -> LN
  "LL -> LN1" : Subsystem  AncestorBlock=|
      | SimplusGT/Grid-Forming Inverter
      | (Simulink Block)/LCL Filter/LL -> LN
  Mux{,1..4} (5 alike) : Mux  Inputs=3
  Three-Phase Series RLC Branch : powerlib/Elements/Three-Phase Series RLC Branch  LConnTagsString=A|B|C  RConnTagsString=A|B|C  BranchType=RL  Resistance=Rf  Inductance=Lf  Capacitance=1e-6  Measurements=None
  Three-Phase Series RLC Branch1 : powerlib/Elements/Three-Phase Series RLC Branch  LConnTagsString=A|B|C  RConnTagsString=A|B|C  BranchType=RL  Resistance=Rc  Inductance=Lc  Capacitance=1e-6  Measurements=None
  Three-Phase Series RLC Branch2 : powerlib/Elements/Three-Phase Series RLC Branch  LConnTagsString=A|B|C  RConnTagsString=A|B|C  BranchType=RC  Resistance=Rd  Inductance=Lc  Capacitance=Cf  Measurements=None
  Vab : powerlib/Measurements/Voltage Measurement  PhasorSimulation=off  OutputType=Complex  PSBequivalent=0
  Vab1 : powerlib/Measurements/Voltage Measurement  PhasorSimulation=off  OutputType=Complex  PSBequivalent=0
  Vbc : powerlib/Measurements/Voltage Measurement  PhasorSimulation=off  OutputType=Complex  PSBequivalent=0
  Vbc1 : powerlib/Measurements/Voltage Measurement  PhasorSimulation=off  OutputType=Complex  PSBequivalent=0
  Vca : powerlib/Measurements/Voltage Measurement  PhasorSimulation=off  OutputType=Complex  PSBequivalent=0
  Vca1 : powerlib/Measurements/Voltage Measurement  PhasorSimulation=off  OutputType=Complex  PSBequivalent=0
  iga : powerlib/Measurements/Current Measurement  PhasorSimulation=off  OutputType=Complex  PSBequivalent=0
  igb : powerlib/Measurements/Current Measurement  PhasorSimulation=off  OutputType=Complex  PSBequivalent=0
  igc : powerlib/Measurements/Current Measurement  PhasorSimulation=off  OutputType=Complex  PSBequivalent=0
  ila : powerlib/Measurements/Current Measurement  PhasorSimulation=off  OutputType=Complex  PSBequivalent=0
  ilb : powerlib/Measurements/Current Measurement  PhasorSimulation=off  OutputType=Complex  PSBequivalent=0
  ilc : powerlib/Measurements/Current Measurement  PhasorSimulation=off  OutputType=Complex  PSBequivalent=0
  vca measure : powerlib/Measurements/Voltage Measurement  PhasorSimulation=off  OutputType=Complex  PSBequivalent=0
  vcb measure : powerlib/Measurements/Voltage Measurement  PhasorSimulation=off  OutputType=Complex  PSBequivalent=0
  vcc measure : powerlib/Measurements/Voltage Measurement  PhasorSimulation=off  OutputType=Complex  PSBequivalent=0
  via : PMIOPort  Side=Left
  vib : PMIOPort  Port=2  Side=Left
  vic : PMIOPort  Port=3  Side=Left
  vga : PMIOPort  Port=4  Side=Right
  vgb : PMIOPort  Port=5  Side=Right
  vgc : PMIOPort  Port=6  Side=Right
  N : PMIOPort  Port=7  Side=Left
  m : Outport
  wires:
  [igabc] -> Bus Creator/5  "igabc"
  [ilabc] -> Bus Creator/4  "ilabc"
  [vgabc] -> Bus Creator/3  "vgabc"
  [vcabc] -> Bus Creator/2  "vcabc"
  [viabc] -> Bus Creator/1  "viabc"
  "LL -> LN"/1(Out1) -> [viabc]
  Vab1/1 -> Mux1/1
  Mux1/1 -> "LL -> LN"/1(In1)
  Vca1/1 -> Mux1/3
  Vbc1/1 -> Mux1/2
  Mux3/1 -> [vcabc]
  "LL -> LN1"/1(Out1) -> [vgabc]
  Bus Creator/1 -> m/1
  Mux2/1 -> [ilabc]
  Vbc/1 -> Mux/2
  ilc/1 -> Mux2/3
  Vca/1 -> Mux/3
  iga/1 -> Mux4/1
  igb/1 -> Mux4/2
  vcb measure/1 -> Mux3/2
  vca measure/1 -> Mux3/1
  Mux/1 -> "LL -> LN1"/1(In1)
  Vab/1 -> Mux/1
  vcc measure/1 -> Mux3/3
  igc/1 -> Mux4/3
  ila/1 -> Mux2/1
  ilb/1 -> Mux2/2
  Mux4/1 -> [igabc]
  connections:
  Three-Phase Series RLC Branch/RConn3 -- ilc/LConn1
  Three-Phase Series RLC Branch/RConn2 -- ilb/LConn1
  Three-Phase Series RLC Branch/RConn1 -- ila/LConn1
  Three-Phase Series RLC Branch1/RConn3 -- igc/LConn1
  Three-Phase Series RLC Branch1/RConn1 -- iga/LConn1
  vga/RConn1 -- iga/RConn1 -- Vca/LConn2 -- Vab/LConn1
  Three-Phase Series RLC Branch2/LConn1 -- vca measure/LConn1 -- Three-Phase Series RLC Branch1/LConn1 -- ila/RConn1
  Three-Phase Series RLC Branch2/LConn2 -- vcb measure/LConn1 -- Three-Phase Series RLC Branch1/LConn2 -- ilb/RConn1
  vgb/RConn1 -- igb/RConn1 -- Vab/LConn2 -- Vbc/LConn1
  Three-Phase Series RLC Branch1/RConn2 -- igb/LConn1
  vcc measure/LConn1 -- Three-Phase Series RLC Branch2/LConn3 -- ilc/RConn1 -- Three-Phase Series RLC Branch1/LConn3
  Three-Phase Series RLC Branch/LConn1 -- via/RConn1 -- Vca1/LConn2 -- Vab1/LConn1
  vib/RConn1 -- Vab1/LConn2 -- Vbc1/LConn1 -- Three-Phase Series RLC Branch/LConn2
  Three-Phase Series RLC Branch/LConn3 -- vic/RConn1 -- Vbc1/LConn2 -- Vca1/LConn1
  vgc/RConn1 -- igc/RConn1 -- Vbc/LConn2 -- Vca/LConn1
  vcb measure/LConn2 -- vca measure/LConn2 -- vcc measure/LConn2 -- Three-Phase Series RLC Branch2/RConn3 -- N/RConn1 -- Three-Phase Series RLC Branch2/RConn2 -- Three-Phase Series RLC Branch2/RConn1

== system SimplusGT_2015a/Grid-Forming Inverter (Simulink Block)/PQ Calculation (dq-Frame) ==
  note: Power calculation.
      |
      | Author(s): Yitong Li
      |
      | Notes:
      |
      | The calculation is done in dq frame.
  vdq : Inport
  idq : Inport  Port=2
  Mux : Mux  Inputs=2
  Mux1 : Mux  Inputs=2
  P = vd*id+vq*iq : Fcn  Expr=u[1]*u[3]+u[2]*u[4]
  Q = -vd*iq+vq*id : Fcn  Expr=-u[1]*u[4]+u[2]*u[3]
  pq : Outport
  wires:
  Mux/1 -> pq/1
  P = vd*id+vq*iq/1 -> Mux/1
  vdq/1 -> Mux1/1
  idq/1 -> Mux1/2
  Mux1/1 -> P = vd*id+vq*iq/1, Q = -vd*iq+vq*id/1
  Q = -vd*iq+vq*id/1 -> Mux/2

== system SimplusGT_2015a/Grid-Forming Inverter (Simulink Block)/Voltage Controller ==
  vcdq* : Inport
  vcdq : Inport  Port=2
  igdq : Inport  Port=3
  enable : Inport  Port=4
  Constant : Constant  Value=Kcd
  Demux1 : Demux  Outputs=2
  Demux2 : Demux  Outputs=2
  Demux3 : Demux  Outputs=2
  Mux : Mux  Inputs=2
  PI-DT-Estimated d : Subsystem  mask{Kg=Kg, Kp=Kp, Ki=Ki, xmax=xdmax, xmin=-xdmax, Ts=Ts}
      mask prompts: Kg "Estimator Gain"; Kp "Proportional Gain"; Ki "Integral Gain"; xmax "Upper Limit"; xmin "Lower Limit"; Ts "Sampling Time"
  PI-DT-Estimated q : Subsystem  mask{Kg=Kg, Kp=Kp, Ki=Ki, xmax=xqmax, xmin=-xqmax, Ts=Ts}
      mask prompts: Kg "Estimator Gain"; Kp "Proportional Gain"; Ki "Integral Gain"; xmax "Upper Limit"; xmin "Lower Limit"; Ts "Sampling Time"
  Product : Product
  Product1 : Product
  sum_d : Sum  Inputs=+-
  sum_q : Sum
  wCd : Gain  Gain=Wbase*Cf
  wCq : Gain  Gain=Wbase*Cf
  ildq* : Outport
  wires:
  sum_d/1 -> Mux/1
  sum_q/1 -> Mux/2
  vcdq/1 -> Demux1/1
  Demux1/1 -> wCd/1, PI-DT-Estimated d/4(actual)
  Demux1/2 -> PI-DT-Estimated q/1(actual), wCq/1
  Mux/1 -> ildq*/1
  PI-DT-Estimated d/1(Out) -> sum_d/1
  igdq/1 -> Demux3/1
  PI-DT-Estimated q/1(Out) -> sum_q/2
  Demux3/2 -> PI-DT-Estimated q/2(initial)
  Demux3/1 -> PI-DT-Estimated d/3(initial)
  vcdq*/1 -> Demux2/1
  Demux2/1 -> PI-DT-Estimated d/2(reference)
  Demux2/2 -> PI-DT-Estimated q/3(reference)
  enable/1 -> PI-DT-Estimated q/4(enable), PI-DT-Estimated d/1(enable)
  wCd/1 -> Product/1
  Product/1 -> sum_q/1
  wCq/1 -> Product1/2
  Product1/1 -> sum_d/2
  Constant/1 -> Product/2, Product1/1

== system SimplusGT_2015a/Grid-Forming Inverter (Simulink Block)/abc -> dq (Power-Invariant) ==
  note: Frame transformation from abc to dq.
      |
      | Author(s): Yitong Li
      |
      | Notes:
      |
      | The transformation is power-invariant.
      |
      | theta is the angle that d axis leads a axis.
      |
      | q axis leads d axis by 90 degrees.
  abc : Inport
  theta : Inport  Port=2
  ->d : Fcn  Expr=cos(u(4))*u(1) + cos(u(4)-2/3*pi)*u(2) + cos(u(4)-4/3*pi)*u(3)
  ->q : Fcn  Expr=-sin(u(4))*u(1) - sin(u(4)-2/3*pi)*u(2) - sin(u(4)-4/3*pi)*u(3)
  Gain : Gain  Gain=sqrt(2/3)
  Mux5 : Mux  Inputs=2
  Mux6 : Mux  Inputs=2
  dq : Outport
  wires:
  abc/1 -> Gain/1
  ->d/1 -> Mux6/1
  Gain/1 -> Mux5/1
  theta/1 -> Mux5/2
  ->q/1 -> Mux6/2
  Mux6/1 -> dq/1
  Mux5/1 -> ->d/1, ->q/1

== system SimplusGT_2015a/Grid-Forming Inverter (Simulink Block)/abc -> dq (Power-Invariant)1 ==
  note: Frame transformation from abc to dq.
      |
      | Author(s): Yitong Li
      |
      | Notes:
      |
      | The transformation is power-invariant.
      |
      | theta is the angle that d axis leads a axis.
      |
      | q axis leads d axis by 90 degrees.
  abc : Inport
  theta : Inport  Port=2
  ->d : Fcn  Expr=cos(u(4))*u(1) + cos(u(4)-2/3*pi)*u(2) + cos(u(4)-4/3*pi)*u(3)
  ->q : Fcn  Expr=-sin(u(4))*u(1) - sin(u(4)-2/3*pi)*u(2) - sin(u(4)-4/3*pi)*u(3)
  Gain : Gain  Gain=sqrt(2/3)
  Mux5 : Mux  Inputs=2
  Mux6 : Mux  Inputs=2
  dq : Outport
  wires:
  abc/1 -> Gain/1
  ->d/1 -> Mux6/1
  Gain/1 -> Mux5/1
  theta/1 -> Mux5/2
  ->q/1 -> Mux6/2
  Mux6/1 -> dq/1
  Mux5/1 -> ->d/1, ->q/1
